simulink model "ecu2vib"  (R2013a)
settings: Solver=ode45  StartTime=0.0  StopTime=400  FixedStep=.01  RelTol=1e-3
undefined symbols (not defined in the file or in its folder): P, S
settings Model: Creator=Daniel  LastModifiedBy=Daniel
settings OptimizationCC: ExpressionDepthLimit=2147483647
settings DebuggingCC: SolverPrmCheckMsg=none

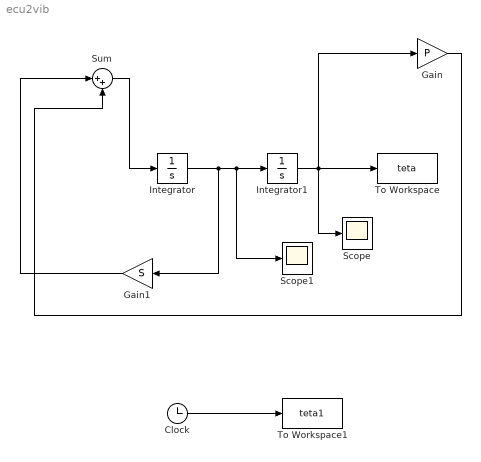
== system ecu2vib ==
  Clock : Clock
  Gain : Gain  Gain=P
  Gain1 : Gain  Gain=S
  Integrator : Integrator
  Integrator1 : Integrator  InitialCondition=pi
  Scope : Scope
      settings: TimeRange=10  YMin=0  YMax=120
  Scope1 : Scope
  Sum : Sum  Inputs=|++
  To Workspace : ToWorkspace  VariableName=teta  SampleTime=-1
  To Workspace1 : ToWorkspace  VariableName=teta1  SampleTime=-1
  wires:
  Integrator1/1 -> Gain/1, To Workspace/1, Scope/1
  Integrator/1 -> Gain1/1, Scope1/1, Integrator1/1
  Gain/1 -> Sum/2
  Clock/1 -> To Workspace1/1
  Gain1/1 -> Sum/1
  Sum/1 -> Integrator/1
